simulink library "dsp_blocks"  (Simulink 10.3)
settings: Solver=VariableStepAuto  StartTime=0.0  StopTime=10.0  RelTol=1e-3
values from neighbouring files (symbols this model uses):
  a = [a1]    [loop_filter1.m]    (also in sfunpsd2.m = [(1:npts)'/npts ones(npts,1)])
  b = [b0 b1]    [loop_filter1.m]
undefined symbols (not defined in the file or in its folder): bits_to_symb_do, DiscIntNeverNeededParam, do_wait, final_delay, input_stream_sample, j, lookup_do, offset, sfunpsd2
libraries: $bdroot x3, simulink x2
settings Model: Creator=jon  LastModifiedBy=adityaojha  ExtModeAutoUpdateStatusClock=off

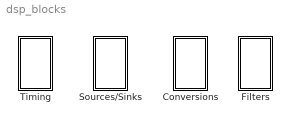
== system dsp_blocks ==
  Conversions : Subsystem
  Filters : Subsystem
  Sources/Sinks : Subsystem
  "Timing " : Subsystem

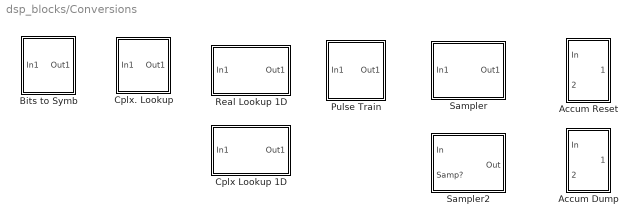
== system dsp_blocks/Conversions ==
  Accum Dump : Subsystem  mask{val0=0}
      mask prompts: val0 "Initial Condition"
      mask help: Accumulate and dump operation.
  Accum Reset : Subsystem
      mask help: Accumulator that can be reset.
  Bits to Symb : Subsystem
      mask help: Converts bits to symbols.
  Cplx Lookup 1D : Subsystem  mask{table=[j -j]}
      mask init:
      | XData = [0:length(table)-1]; YDataRe = real(table); YDataIm = imag(table); XDataEvenlySpacing=1;
  Cplx. Lookup : Subsystem  mask{table=[-1 1]}
      mask help: Does a discrete lookup table.
      mask Help: The table variable has one entry per possible input index.  Note that it is defined to be zero indexed (0 maps to the first table entry, 1 to the second, etc.).
  Pulse Train : Subsystem  mask{period=10}
      mask prompts: period "Period (samples)"
      mask help: Samples the incoming signal and makes a pulse train.
      mask Display: disp(sprintf('T=%d', period));
  Real Lookup 1D : Subsystem  mask{table=[-1 -0.5 0.5 1]}
      mask init:
      | XData = [0:length(table)-1]; YData = table; XDataEvenlySpacing=1;
  Sampler : Subsystem  mask{offset=64, samp_period=10}
      mask prompts: offset "Offset (samples)"; samp_period "Sample Period"
      mask Display: disp(sprintf('del=%d, T=%d', offset, samp_period));
  Sampler2 : Subsystem
      mask help: Sample and hold with external gate signal.

== system dsp_blocks/Filters ==
  RC FIR Filter : Subsystem  mask{period=10, beta=0.5, root=off, filt_len=128, win_type=off}
      mask prompts: period "Symbol Period"; beta "Roll Off (beta)"; root "Root Filter?"; filt_len "Filter Length (taps)"; win_type "Hamming Window?"
      mask init:
      | symb_rate = 1/period; p.fs = symb_rate; p.beta = beta; p.root = root; [h f Ha Hi win] = win_method('rc_filt', p, 1.5*(1+beta)*symb_rate, 1, filt_len, win_type); h = h';
      mask Display: plot(f, abs(Ha));
  RECT Filter : Subsystem  AncestorBlock=dsp_blocks/Filters/RC FIR Filter  mask{f0=0.1, f1=0.2, filt_len=64}
      mask prompts: f0 "Low Cutoff (0=LPF)"; f1 "Hi Cutoff"; filt_len "Filter Length (taps)"
      mask init:
      | p.x1 = f0; p.x2 = f0; p.x3 = f1; p.x4 = f1; [h f Ha Hi win] = win_method('pw_lin', p, 0.5, 1, filt_len, 1); h = h';
      mask Display: plot(f, abs(Ha));

== system dsp_blocks/Sources/Sinks ==
  Averaging Power Spectral Density dB : Subsystem  LoadFcn=sfunpsd2([],[],[],'LoadBlock')  StartFcn=sfunpsd2([],[],[],'Start')  mask(Spectrum Analyzer){npts=128, fftpts=512, HowOften=64, sampleT=1, db_range=20}
      mask prompts: npts "Length of buffer:"; fftpts "Number of points for fft:"; HowOften "Plot after how many points:"; sampleT "Sample time:"; db_range "dB Range:"
      mask help: Spectrum analyzer using graph window.
      mask init:
      | ts=sampleT(1); if length(sampleT) > 1, offset = sampleT(2);, else, offset = 0; end
      settings: CopyFcn=sfunpsd2([],[],[],'CopyBlock')  DeleteFcn=sfunpsd2([],[],[],'DeleteBlock')  NameChangeFcn=sfunpsd2([],[],[],'NameChange')
      mask Help: This block when hooked to the output of a system displays the frequency content of the buffer in the graph window. For more see the M-file sfunpsd.
      mask Display: plot(0,0,100,100,[11,92,92,11,11],[90,90,40,40,90],[82,76,65,57,51,44,35,30,25,20],[65,62,59,63,66,66,67,70,55,50])
  Input Stream : Subsystem  mask{period=10, width=1, fname=data.mat}
      mask prompts: fname "Data Filename"
      mask help: Input Stream: Reads binary data from an input file. Outputs a new value once per period. Width allows you to multiplex output.
      mask init:
      | load(fname); N = floor(length(data)/width); data = reshape(data(1:N*width),width,N);
      mask Help: The function loads the binary data from file fname, which should have a single vector called "data".  The output of the block is updated once every T=width*period.
      mask Display: disp(sprintf('file=%s\nT=%g w=%d', fname, period, width))

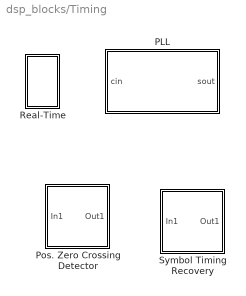
== system dsp_blocks/Timing  ==
  PLL : Subsystem  mask{freq=0.1, freq_out=0.1, phi=0, amp=1, xi=1, K=2, T=200}
      mask prompts: freq "Input Frequency"; freq_out "Output Frequency"; phi "Output Phase"; amp "Output Amplitude"; xi "Damping Factor"; K "Loop Gain"; T "Loop Time Constant (samples)"
      mask help: Implements a phase locked loop (PLL).
      mask init:
      | [a, b, tau1, tau2, Kout] = loop_filter1(T, xi, K);
      mask Display: disp(sprintf('fin=%g fout=%g\nxi=%g Tl=%g\nphi=%g  amp=%g',freq,freq_out,xi,T,phi,amp));
  Pos. Zero Crossing Detector : Subsystem
      mask help: Detects a positive slope zero crossing.
  Real-Time : Subsystem  mask{scale=1}
      mask prompts: scale "Scale Factor"
      mask help: This block slows down a simulation so sample time is some fraction of the real time.
      mask Display: disp('RT');
  Symbol Timing Recovery : Subsystem  mask{T=50, Tl=1000, tadj=0}
      mask prompts: T "Symbol Period"; Tl "PLL Time Constant (samples)"; tadj "Timing Adjust"
      mask help: Symbol Timing Recovery Block
      mask init:
      | if (tadj < 0), final_delay=T+tadj; else final_delay=tadj; end
      mask Display: disp(sprintf('T=%g\nTl=%g\ntadj=%g\n', T, Tl,tadj));

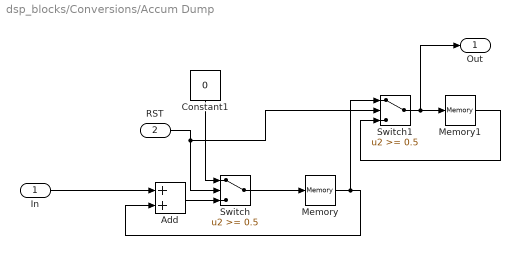
== system dsp_blocks/Conversions/Accum Dump ==
  In : Inport
  RST : Inport  Port=2
  Add : Sum
  Constant1 : Constant  Value=0
  Memory : Memory  InitialCondition=val0
  Memory1 : Memory  InitialCondition=val0
  Switch : Switch  Threshold=0.5
  Switch1 : Switch  Threshold=0.5
  Out : Outport
  wires:
  Switch/1 -> Memory/1
  Add/1 -> Switch/3
  RST/1 -> Switch/2, Switch1/2
  Constant1/1 -> Switch/1
  In/1 -> Add/1
  Memory/1 -> Add/2, Switch1/1
  Switch1/1 -> Memory1/1, Out/1
  Memory1/1 -> Switch1/3

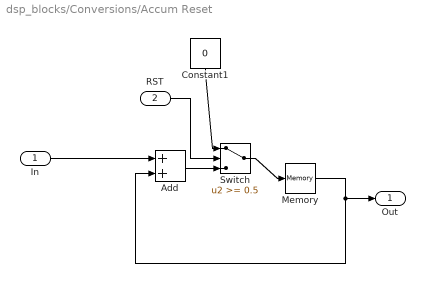
== system dsp_blocks/Conversions/Accum Reset ==
  In : Inport
  RST : Inport  Port=2
  Add : Sum
  Constant1 : Constant  Value=0
  Memory : Memory
  Switch : Switch  Threshold=0.5
  Out : Outport
  wires:
  Switch/1 -> Memory/1
  Memory/1 -> Add/2, Out/1
  Add/1 -> Switch/3
  RST/1 -> Switch/2
  Constant1/1 -> Switch/1
  In/1 -> Add/1

== system dsp_blocks/Conversions/Bits to Symb ==
  In1 : Inport
  MATLAB Fcn : MATLABFcn  MATLABFcn=bits_to_symb_do(u)  OutputDimensions=1
  Out1 : Outport
  wires:
  MATLAB Fcn/1 -> Out1/1
  In1/1 -> MATLAB Fcn/1

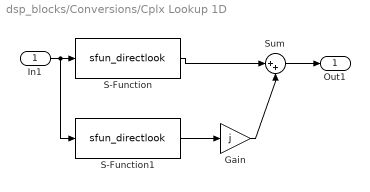
== system dsp_blocks/Conversions/Cplx Lookup 1D ==
  In1 : Inport
  Gain : Gain  Gain=j  SaturateOnIntegerOverflow=on  OutDataTypeStr=Inherit: Same as input  ParamDataTypeStr=Inherit: Same as input
  S-Function : S-Function  FunctionName=sfun_directlook  Parameters=XData, YDataRe, XDataEvenlySpacing  SFunctionDeploymentMode=off  EnableBusSupport=off
  S-Function1 : S-Function  FunctionName=sfun_directlook  Parameters=XData, YDataIm, XDataEvenlySpacing  SFunctionDeploymentMode=off  EnableBusSupport=off
  Sum : Sum  Inputs=|++  InputSameDT=on  SaturateOnIntegerOverflow=on  OutDataTypeStr=Inherit: Same as first input
  Out1 : Outport
  wires:
  In1/1 -> S-Function1/1, S-Function/1
  S-Function/1 -> Sum/1
  Gain/1 -> Sum/2
  Sum/1 -> Out1/1
  S-Function1/1 -> Gain/1

== system dsp_blocks/Conversions/Cplx. Lookup ==
  In1 : Inport
  MATLAB Fcn : MATLABFcn  MATLABFcn=lookup_do(u, table)  OutputSignalType=complex
  Out1 : Outport
  wires:
  MATLAB Fcn/1 -> Out1/1
  In1/1 -> MATLAB Fcn/1

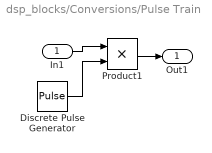
== system dsp_blocks/Conversions/Pulse Train ==
  In1 : Inport
  Discrete Pulse Generator : DiscretePulseGenerator  Period=period
  Product1 : Product  RndMeth=Zero  SaturateOnIntegerOverflow=on  OutDataTypeStr=Inherit: Same as first input
  Out1 : Outport
  wires:
  Product1/1 -> Out1/1
  In1/1 -> Product1/1
  Discrete Pulse Generator/1 -> Product1/2

== system dsp_blocks/Conversions/Real Lookup 1D ==
  In1 : Inport
  S-Function : S-Function  FunctionName=sfun_directlook  Parameters=XData, YData, XDataEvenlySpacing  SFunctionDeploymentMode=off  EnableBusSupport=off
  Out1 : Outport
  wires:
  S-Function/1 -> Out1/1
  In1/1 -> S-Function/1

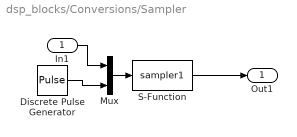
== system dsp_blocks/Conversions/Sampler ==
  In1 : Inport
  Discrete Pulse Generator : DiscretePulseGenerator  Period=samp_period  PhaseDelay=offset
  Mux : Mux  Inputs=2
  S-Function : S-Function  FunctionName=sampler1  SFunctionDeploymentMode=off  EnableBusSupport=off
  Out1 : Outport
  wires:
  S-Function/1 -> Out1/1
  Mux/1 -> S-Function/1
  In1/1 -> Mux/1
  Discrete Pulse Generator/1 -> Mux/2

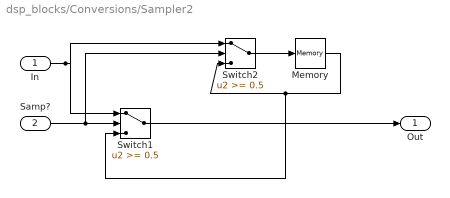
== system dsp_blocks/Conversions/Sampler2 ==
  In : Inport
  Samp? : Inport  Port=2
  Memory : Memory
  Switch1 : Switch  Threshold=0.5
  Switch2 : Switch  Threshold=0.5
  Out : Outport
  wires:
  Samp?/1 -> Switch1/2, Switch2/2
  In/1 -> Switch1/1, Switch2/1
  Switch1/1 -> Out/1
  Switch2/1 -> Memory/1
  Memory/1 -> Switch2/3, Switch1/3

== system dsp_blocks/Filters/RC FIR Filter ==
  In1 : Inport
  Discrete Filter2 : DiscreteFilter  Numerator=h  Denominator=[1]  SampleTime=1
  Out1 : Outport
  wires:
  Discrete Filter2/1 -> Out1/1
  In1/1 -> Discrete Filter2/1

== system dsp_blocks/Filters/RECT Filter ==
  In1 : Inport
  Discrete Filter2 : DiscreteFilter  Numerator=h  Denominator=[1]  SampleTime=1
  Out1 : Outport
  wires:
  In1/1 -> Discrete Filter2/1
  Discrete Filter2/1 -> Out1/1

== system dsp_blocks/Sources/Sinks/Averaging Power Spectral Density dB ==
  input signal : Inport
  sfunpsd2 : S-Function  LoadFcn=sfunpsd2([],[],[],'LoadBlock')  StartFcn=sfunpsd2([],[],[],'Start')  FunctionName=sfunpsd2  Parameters=fftpts,npts,HowOften,offset,ts,1,db_range  SFunctionDeploymentMode=off  EnableBusSupport=off
      settings: CopyFcn=sfunpsd2([],[],[],'CopyBlock')  DeleteFcn=sfunpsd2([],[],[],'DeleteBlock')  NameChangeFcn=sfunpsd2([],[],[],'NameChange')
  wires:
  input signal/1 -> sfunpsd2/1

== system dsp_blocks/Sources/Sinks/Input Stream ==
  Clock : Clock
  MATLAB Fcn : MATLABFcn  MATLABFcn=input_stream_sample(u, data, period, width)  OutputDimensions=width  Output1D=off
  Out1 : Outport
  wires:
  MATLAB Fcn/1 -> Out1/1
  Clock/1 -> MATLAB Fcn/1

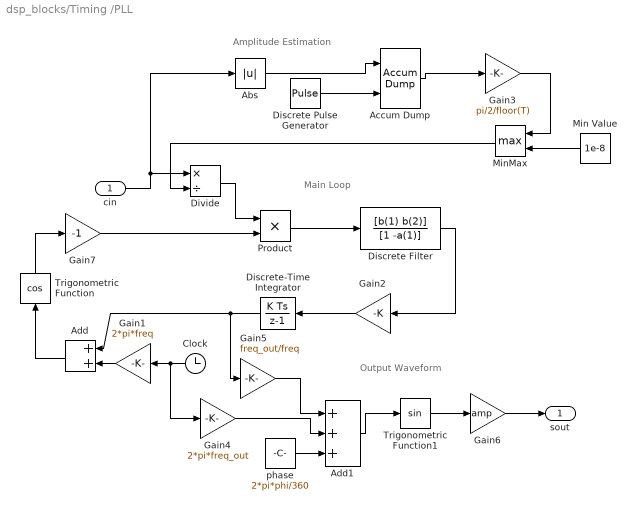
== system dsp_blocks/Timing /PLL ==
  note: Output Waveform
  note: Main Loop
  note: Amplitude Estimation
  cin : Inport
  Abs : Abs
  Accum Dump : $bdroot/Conversions/Accum Dump  val0=2/pi*floor(T)
  Add : Sum
  Add1 : Sum  Inputs=+++
  Clock : Clock
  Discrete Filter : DiscreteFilter  Numerator=[b(1) b(2)]  Denominator=[1 -a(1)]  SampleTime=1
  Discrete Pulse Generator : DiscretePulseGenerator  Period=floor(T)
  Discrete-Time Integrator : DiscreteIntegrator  gainval=1  ICPrevOutput=DiscIntNeverNeededParam  ICPrevScaledInput=DiscIntNeverNeededParam
  Divide : Product  Inputs=*/
  Gain1 : Gain  Gain=2*pi*freq
  Gain2 : Gain  Gain=-K
  Gain3 : Gain  Gain=pi/2/floor(T)
  Gain4 : Gain  Gain=2*pi*freq_out
  Gain5 : Gain  Gain=freq_out/freq
  Gain6 : Gain  Gain=amp
  Gain7 : Gain  Gain=-1
  Min Value : Constant  Value=1e-8
  MinMax : MinMax  Function=max  Inputs=2
  Product : Product  RndMeth=Zero
  Trigonometric Function : Trigonometry  Operator=cos
  Trigonometric Function1 : Trigonometry
  phase : Constant  Value=2*pi*phi/360
  sout : Outport
  wires:
  Trigonometric Function1/1 -> Gain6/1
  Add1/1 -> Trigonometric Function1/1
  Gain5/1 -> Add1/1
  Gain4/1 -> Add1/2
  Min Value/1 -> MinMax/2
  MinMax/1 -> Divide/2
  Gain3/1 -> MinMax/1
  Divide/1 -> Product/1
  cin/1 -> Divide/1, Abs/1
  Abs/1 -> Accum Dump/1
  Discrete Filter/1 -> Gain2/1
  Gain2/1 -> Discrete-Time Integrator/1
  Trigonometric Function/1 -> Gain7/1
  Add/1 -> Trigonometric Function/1
  Discrete-Time Integrator/1 -> Gain5/1, Add/1
  Gain1/1 -> Add/2
  Clock/1 -> Gain4/1, Gain1/1
  Product/1 -> Discrete Filter/1
  Gain6/1 -> sout/1
  Gain7/1 -> Product/2
  phase/1 -> Add1/3
  Accum Dump/1 -> Gain3/1
  Discrete Pulse Generator/1 -> Accum Dump/2

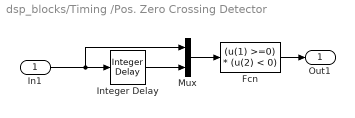
== system dsp_blocks/Timing /Pos. Zero Crossing Detector ==
  In1 : Inport
  Fcn : Fcn  Expr=(u(1) >=0) * (u(2) < 0)
  Integer Delay : simulink/Discrete/Integer Delay  vinit=0.0  samptime=1  NumDelays=1
      settings: SourceProductBaseCode=SL
  Mux : Mux  Inputs=2
  Out1 : Outport
  wires:
  In1/1 -> Integer Delay/1, Mux/1
  Integer Delay/1 -> Mux/2
  Mux/1 -> Fcn/1
  Fcn/1 -> Out1/1

== system dsp_blocks/Timing /Real-Time ==
  Clock : Clock
  MATLAB Fcn : MATLABFcn  Description=do_wait  MATLABFcn=do_wait(u, scale)  OutputDimensions=0
  wires:
  Clock/1 -> MATLAB Fcn/1

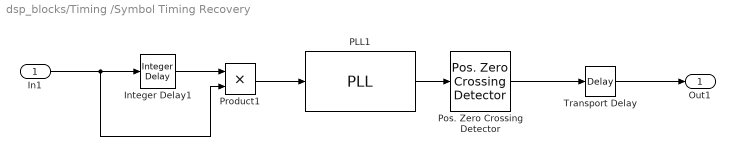
== system dsp_blocks/Timing /Symbol Timing Recovery ==
  In1 : Inport
  Integer Delay1 : simulink/Discrete/Integer Delay  vinit=0.0  samptime=-1  NumDelays=round(T/2)
      settings: SourceProductBaseCode=SL
  PLL1 : $bdroot/Timing /PLL  freq=1/T  freq_out=1/T  phi=0  amp=1  xi=1  K=2  T=Tl
  Pos. Zero Crossing Detector : $bdroot/Timing /Pos. Zero Crossing Detector
  Product1 : Product  RndMeth=Zero
  Transport Delay : TransportDelay  DelayTime=final_delay
  Out1 : Outport
  wires:
  Transport Delay/1 -> Out1/1
  In1/1 -> Integer Delay1/1, Product1/2
  Pos. Zero Crossing Detector/1 -> Transport Delay/1
  PLL1/1 -> Pos. Zero Crossing Detector/1
  Product1/1 -> PLL1/1
  Integer Delay1/1 -> Product1/1
